simulink model "simulink_pd"  (Simulink 8.9)
settings: Solver=FixedStepAuto  StartTime=0.0  StopTime=20  FixedStep=0.1  RelTol=1e-3  EnableMultiTasking=on
values from neighbouring files (symbols this model uses):
  dof = 5    [drone76.m]    (also in link_dynamics.m; result_C curve.mat; result_C_curve.mat; robotarm6_20.m = 3)
  q0 = [0 -pi/2 0 0 0]    [drone76.m]    (also in result_C curve.mat = [0 -1.57079632679 0 0 0]; result_C_curve.mat = [0 -1.57079632679 0 0 0]; robotarm6_20.m = [1e-4 0 pi/6 0 pi/4 0]; test.m)
  q_start = [1e-4 0 1e-4 pi/30 pi/30]    [drone76.m]    (also in result_C curve.mat = [0.0001 0 0.0001 0.10471975512 0.10471975512]; result_C_curve.mat = [0.0001 0 0.0001 0.10471975512 0.10471975512]; test.m)
  xd = [ (1:200)' xb_repro(1,:)']    [drone76.m]    (also in result_C curve.mat = [1 2 3 4 5 6 7 8 9 10 11 12 ... (400 elements, 200x2)]; result_C_curve.mat = [1 2 3 4 5 6 7 8 9 10 11 12 ... (400 elements, 200x2)])
  yaw = yaw-pi    [drone76.m]    (also in result_C curve.mat = [1.80393744259 1.82426283158 1.84411494551 1.86372395965 1.8; result_C_curve.mat = [1.80393744259 1.82426283158 1.84411494551 1.86372395965 1.8)
  zd = [ (1:200)' xb_repro(3,:)']    [drone76.m]    (also in result_C curve.mat = [1 2 3 4 5 6 7 8 9 10 11 12 ... (400 elements, 200x2)]; result_C_curve.mat = [1 2 3 4 5 6 7 8 9 10 11 12 ... (400 elements, 200x2)])
settings Model: Creator=SuseongKim  LastModifiedBy=jbs
settings DataIOCC: SignalLoggingSaveFormat=Dataset
settings OptimizationCC: ExpressionDepthLimit=2147483647
settings DebuggingCC: SolverPrmCheckMsg=warning  FcnCallInpInsideContextMsg=error

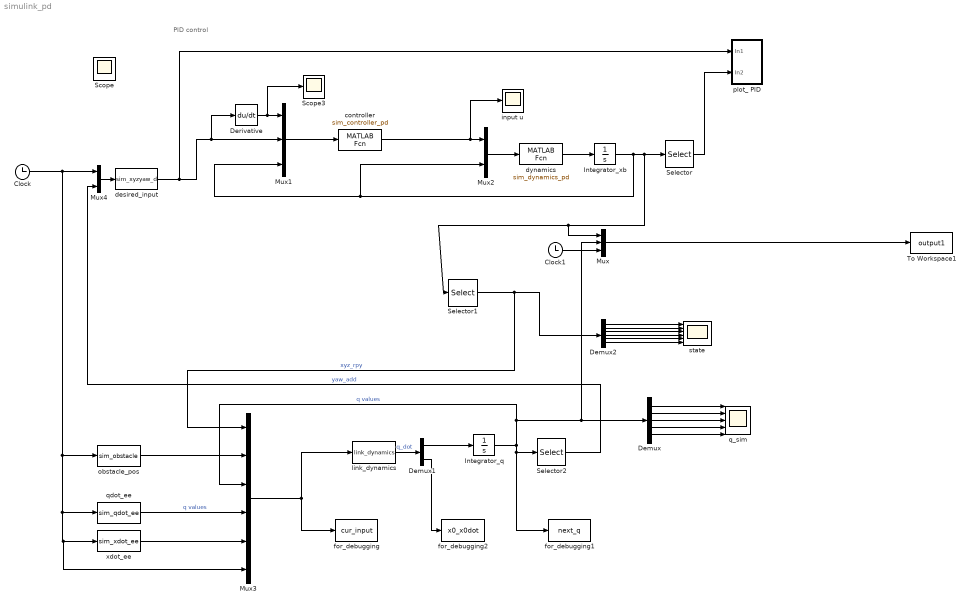
== system simulink_pd ==
  note: PID control
  Clock : Clock
  Clock1 : Clock
  Demux : Demux  Outputs=5
  Demux1 : Demux  Outputs=[5 6]
  Demux2 : Demux  Outputs=6
  Derivative : Derivative
  Integrator_q : Integrator  InitialCondition=q0+q_start  LimitOutput=on
  Integrator_xb : Integrator  InitialCondition="[xd(1,2) 0 zd(1,2)  0 0 yaw(1) 0 0 0 0 0 0]"
  Mux : Mux  Inputs=3
  Mux1 : Mux  Inputs=3
  Mux2 : Mux  Inputs=2
  Mux3 : Mux  Inputs=6
  Mux4 : Mux  Inputs=2
  Scope3 : Scope
  Selector : Selector  InputPortWidth=12  IndexOptions=Index vector (dialog)  Indices=[1 2 3 6]  OutputSizes=1
  Selector1 : Selector  InputPortWidth=12  IndexOptions=Index vector (dialog)  Indices=[1 2 3 4 5 6]  OutputSizes=1
  Selector2 : Selector  InputPortWidth=5  IndexOptions=Index vector (dialog)  Indices=[1]  OutputSizes=1
  To Workspace1 : ToWorkspace  VariableName=output1  SampleTime=-1
  controller : MATLABFcn  MATLABFcn=sim_controller_pd  OutputDimensions=4
  desired_input : MATLABFcn  MATLABFcn=sim_xyzyaw_d  OutputDimensions=4
  dynamics : MATLABFcn  MATLABFcn=sim_dynamics_pd  OutputDimensions=12
  for_debugging : ToWorkspace  VariableName=cur_input  SaveFormat=Timeseries  SampleTime=-1
  for_debugging1 : ToWorkspace  VariableName=next_q  SaveFormat=Timeseries  SampleTime=-1
  for_debugging2 : ToWorkspace  VariableName=x0_x0dot  SaveFormat=Timeseries  SampleTime=-1
  input u : Scope
  link_dynamics : MATLABFcn  MATLABFcn=link_dynamics  OutputDimensions=dof+6
  obstacle_pos : MATLABFcn  MATLABFcn=sim_obstacle  OutputDimensions=3
  plot_ PID : Subsystem
  "q_sim " : Scope  NumInputPorts=5
  qdot_ee : MATLABFcn  MATLABFcn=sim_qdot_ee  OutputDimensions=5
  "state " : Scope  NumInputPorts=6
  xdot_ee : MATLABFcn  MATLABFcn=sim_xdot_ee  OutputDimensions=3
  Scope : Scope
  wires:
  dynamics/1 -> Integrator_xb/1
  Mux1/1 -> controller/1
  Derivative/1 -> Scope3/1, Mux1/1
  Clock/1 -> Mux3/6, xdot_ee/1, qdot_ee/1, obstacle_pos/1, Mux4/1
  Mux2/1 -> dynamics/1
  controller/1 -> Mux2/1, input u/1
  Integrator_xb/1 -> Mux2/2, Mux1/3, Selector/1, Mux/1, Selector1/1
  Demux2/1 -> "state "/1
  Demux2/2 -> "state "/2
  Demux2/3 -> "state "/3
  Demux2/4 -> "state "/4
  Demux2/5 -> "state "/5
  Demux2/6 -> "state "/6
  Selector1/1 -> Mux3/1, Demux2/1  "xyz_rpy"
  Clock1/1 -> Mux/3
  Mux/1 -> To Workspace1/1
  obstacle_pos/1 -> Mux3/2
  Integrator_q/1 -> for_debugging1/1, Selector2/1, Mux3/3, Mux/2, Demux/1  "q values"
  Mux4/1 -> desired_input/1
  Selector2/1 -> Mux4/2  "yaw_add"
  xdot_ee/1 -> Mux3/5
  Mux3/1 -> link_dynamics/1, for_debugging/1
  desired_input/1 -> plot_ PID/1(In1), Mux1/2, Derivative/1
  Selector/1 -> plot_ PID/2(In2)
  Demux/1 -> "q_sim "/1
  Demux/2 -> "q_sim "/2
  Demux/3 -> "q_sim "/3
  Demux/4 -> "q_sim "/4
  Demux/5 -> "q_sim "/5
  qdot_ee/1 -> Mux3/4  "q values"
  Demux1/1 -> Integrator_q/1
  link_dynamics/1 -> Demux1/1  "q_dot"
  Demux1/2 -> for_debugging2/1

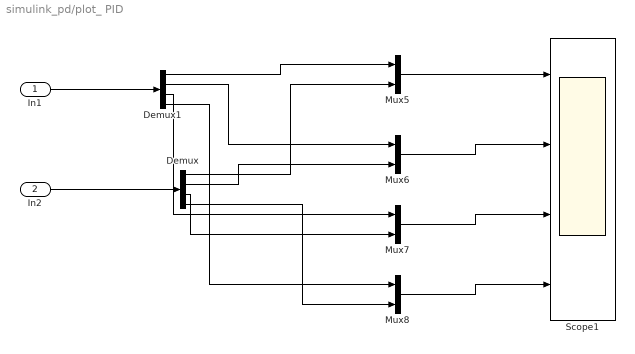
== system simulink_pd/plot_ PID ==
  In1 : Inport
  In2 : Inport  Port=2
  Demux : Demux
  Demux1 : Demux
  Mux{5..8} (4 alike) : Mux  Inputs=2
  Scope1 : Scope  NumInputPorts=4
  wires:
  Demux/1 -> Mux5/2
  Demux/2 -> Mux6/2
  Demux1/4 -> Mux8/1
  Demux1/1 -> Mux5/1
  Demux/4 -> Mux8/2
  Demux1/3 -> Mux7/1
  Demux/3 -> Mux7/2
  Demux1/2 -> Mux6/1
  Mux8/1 -> Scope1/4
  Mux5/1 -> Scope1/1
  In1/1 -> Demux1/1
  Mux7/1 -> Scope1/3
  Mux6/1 -> Scope1/2
  In2/1 -> Demux/1
